simulink model "zaj_3_rt"  (R2015a)
settings: Solver=ode4  StartTime=0.0  StopTime=300  FixedStep=0.1  RelTol=1e-3
settings Model: Creator=Student  LastModifiedBy=lenovo
settings DataIOCC: InspectSignalLogs=on

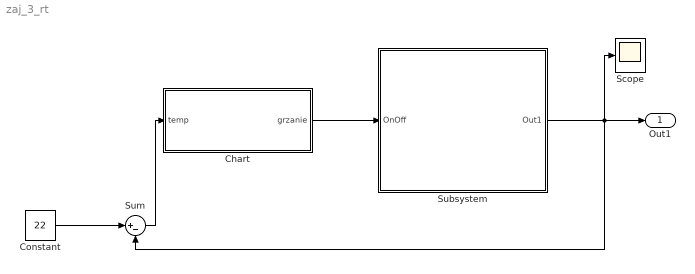
== system zaj_3_rt ==
  Chart : Stateflow chart  TreatAsAtomicUnit=on
  Constant : Constant  Value=22
  Scope : Scope
      settings: TickLabels=on  TimeRange=600  YMax=25  SaveName=ScopeData2
  Subsystem : Subsystem
  Sum : Sum  Inputs=|+-
  Out1 : Outport
  wires:
  Subsystem/1(Out1) -> Out1/1, Sum/2, Scope/1
  Constant/1 -> Sum/1
  Sum/1 -> Chart/1(temp)
  Chart/1(grzanie) -> Subsystem/1(OnOff)

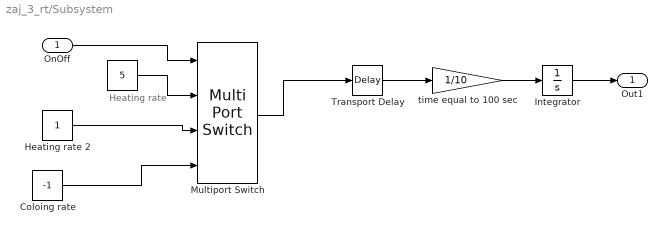
== system zaj_3_rt/Subsystem ==
  note: Heating rate
  OnOff : Inport
  " " : Constant  Value=5
  " Heating rate 2" : Constant
  Coloing rate : Constant  Value=-1
  Integrator : Integrator
  Multiport Switch : MultiPortSwitch  DataPortOrder=Zero-based contiguous
  Transport Delay : TransportDelay
  time equal to 100 sec : Gain  Gain=1/10
  Out1 : Outport
  wires:
  time equal to 100 sec/1 -> Integrator/1
  Transport Delay/1 -> time equal to 100 sec/1
  Integrator/1 -> Out1/1
  Multiport Switch/1 -> Transport Delay/1
  OnOff/1 -> Multiport Switch/1
  " "/1 -> Multiport Switch/2
  " Heating rate 2"/1 -> Multiport Switch/3
  Coloing rate/1 -> Multiport Switch/4

== stateflow chart zaj_3_rt/Chart ==
  state Onmain
    state Heating1 [parallel]
      settings: executionOrder=1
      state On
      state Off
      Onmain.Heating1.On -> Onmain.Heating1.Off : [temp>3]
      (default) -> Onmain.Heating1.Off
      Onmain.Heating1.Off -> Onmain.Heating1.On : [temp<=3]
    state Heating2 [parallel]
      settings: executionOrder=2
      state On
      state Off
      Onmain.Heating2.On -> Onmain.Heating2.Off : [temp>0]
      (default) -> Onmain.Heating2.Off
      Onmain.Heating2.Off -> Onmain.Heating2.On : [temp<0]
    state Heating [parallel]
      during:grzanie=in(Heating1.On)+in(Heating2.On);
      settings: executionOrder=3
  data: temp input; grzanie output
